simulink model "Simulink concentración de tanques"  (R2018a)
settings: Solver=VariableStepAuto  StartTime=0.0  StopTime=90  RelTol=1e-3
settings Model: Creator=ESTUDIANTE  LastModifiedBy=ESTUDIANTE

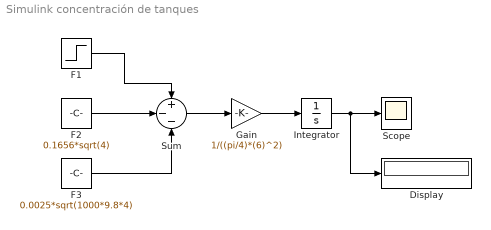
== system Simulink concentración de tanques ==
  Display : Display
  F1 : Step  Before=4  After=4+4*0.1  SampleTime=0
  "F2 " : Constant  Value=0.1656*sqrt(4)
  F3 : Constant  Value=0.0025*sqrt(1000*9.8*4)
  Gain : Gain  Gain=1/((pi/4)*(6)^2)
  Integrator : Integrator  InitialCondition=4
  Scope : Scope
  Sum : Sum  Inputs=+--
  wires:
  F1/1 -> Sum/1
  "F2 "/1 -> Sum/2
  F3/1 -> Sum/3
  Sum/1 -> Gain/1
  Gain/1 -> Integrator/1
  Integrator/1 -> Display/1, Scope/1
